simulink model "testTrigger"  (R2016a)
settings: Solver=VariableStepAuto  StartTime=0.0  StopTime=10.0  RelTol=1e-3
settings Model: Creator=xingye  LastModifiedBy=xingye

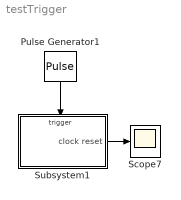
== system testTrigger ==
  Pulse Generator1 : DiscretePulseGenerator  PulseType=Time based  Period=0.1  PulseWidth=5  PhaseDelay=.001
  Scope7 : Scope
  Subsystem1 : Subsystem
  wires:
  Pulse Generator1/1 -> Subsystem1/Trigger
  Subsystem1/1(clock reset) -> Scope7/1

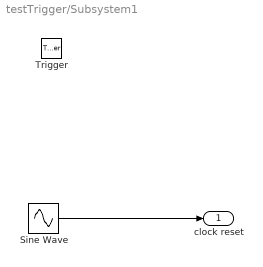
== system testTrigger/Subsystem1 ==
  Trigger : TriggerPort  VariantControl=Variant  PortDimensions=1
  Sine Wave : Sin  Phase=pi/4
  clock reset : Outport
  wires:
  Sine Wave/1 -> clock reset/1
